simulink model "rocket"  (R2023a)
settings: Solver=ode4  StartTime=0.0  StopTime=t  FixedStep=1/24  RelTol=1e-3
values from neighbouring files (symbols this model uses):
  F_min = F_th / 4    (= 211250)    [rocket_sim.m]
  F_th = 845000    [rocket.m]    (also in rocket_sim.m)
  g = 9.81    [rocket_sim.m]
  h0 = 10000    [rocket.m]    (also in rocket_sim.m)
  h_ref = -1    [rocket_sim.m]
  k = 5.47    [rocket.m]    (also in rocket_sim.m)
  Kd = 1    [rocket.m]    (also in rocket_sim.m = 125000)
  Ki = 1    [rocket.m]    (also in rocket_sim.m = 20000)
  Kp = 1    [rocket.m]    (also in rocket_sim.m = 100000)
  m = 25000    [rocket.m]    (also in rocket_sim.m)
  v_term = -211    [rocket.m]    (also in rocket_sim.m)
settings Model: Creator=eriknymobohne  LastModifiedBy=eriknymobohne

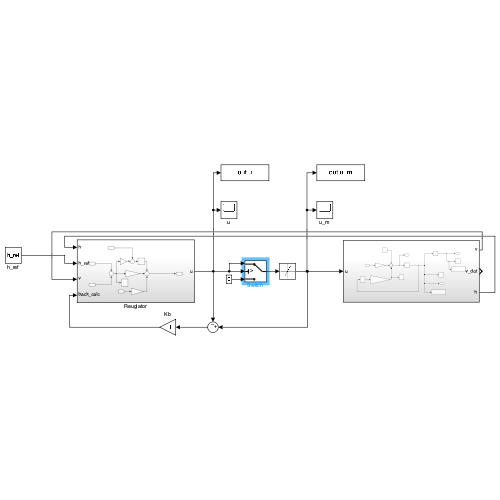
[thumbnail: Simulink's stored preview of the top-level diagram]
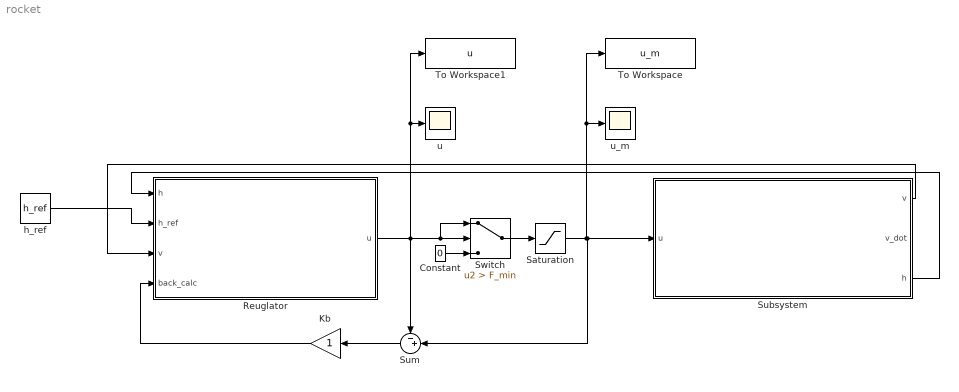
== system rocket ==
  Constant : Constant  Value=0
  Kb : Gain
  Reuglator : Subsystem
  Saturation : Saturate  UpperLimit=F_th  LowerLimit=0
  Subsystem : Subsystem
  Sum : Sum  Inputs=-+|
  Switch : Switch  Criteria=u2 > Threshold  Threshold=F_min  SaturateOnIntegerOverflow=off  InputSameDT=off
  To Workspace : ToWorkspace  VariableName=u_m  SaveFormat=Timeseries  SampleTime=-1
  To Workspace1 : ToWorkspace  VariableName=u  SaveFormat=Timeseries  SampleTime=-1
  h_ref : Constant  Value=h_ref
  u : Scope
  u_m : Scope
  wires:
  h_ref/1 -> Reuglator/2(h_ref)
  Reuglator/1(u) -> Switch/1, Switch/2, To Workspace1/1, u/1, Sum/1
  Saturation/1 -> To Workspace/1, u_m/1, Sum/2, Subsystem/1(u)
  Sum/1 -> Kb/1
  Kb/1 -> Reuglator/4(back_calc)
  Subsystem/3(h) -> Reuglator/1(h)
  Subsystem/1(v) -> Reuglator/3(v)
  Switch/1 -> Saturation/1
  Constant/1 -> Switch/3

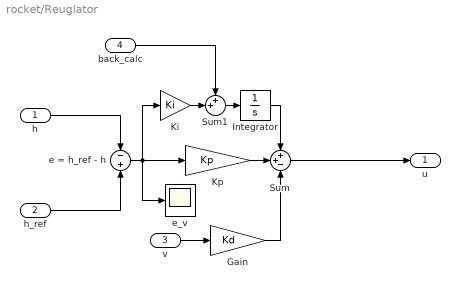
== system rocket/Reuglator ==
  h : Inport
  h_ref : Inport  Port=2
  v : Inport  Port=3
  back_calc : Inport  Port=4
  Gain : Gain  Gain=Kd
  Integrator : Integrator
  Ki : Gain  Gain=Ki
  Kp : Gain  Gain=Kp
  Sum : Sum  Inputs=++-
  Sum1 : Sum  Inputs=++|
  e = h_ref - h : Sum  Inputs=-|+
  e_v : Scope
  u : Outport
  wires:
  h_ref/1 -> e = h_ref - h/2
  h/1 -> e = h_ref - h/1
  e = h_ref - h/1 -> e_v/1, Ki/1, Kp/1
  Kp/1 -> Sum/2
  Integrator/1 -> Sum/1
  v/1 -> Gain/1
  Ki/1 -> Sum1/2
  Sum1/1 -> Integrator/1
  Sum/1 -> u/1
  back_calc/1 -> Sum1/1
  Gain/1 -> Sum/3

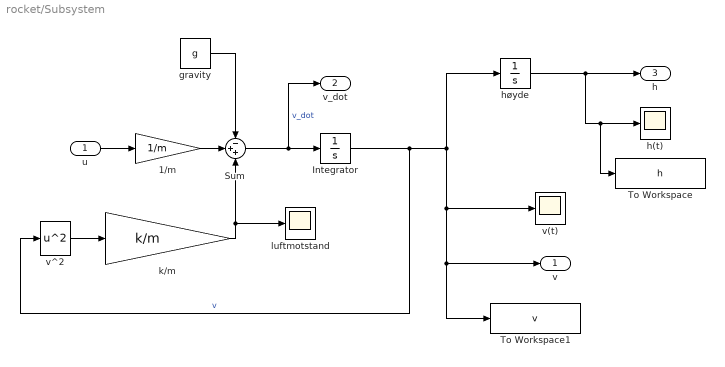
== system rocket/Subsystem ==
  u : Inport
  1/m : Gain  Gain=1/m
  Integrator : Integrator  InitialCondition=v_term
  Sum : Sum  Inputs=-++
  To Workspace : ToWorkspace  VariableName=h  SaveFormat=Timeseries  SampleTime=-1
  To Workspace1 : ToWorkspace  VariableName=v  SaveFormat=Timeseries  SampleTime=-1
  gravity : Constant  Value=g
  h(t) : Scope
  høyde : Integrator  InitialCondition=h0
  k/m : Gain  Gain=k/m
  luftmotstand : Scope
  v(t) : Scope
  v^2 : Math  Operator=square
  v : Outport
  v_dot : Outport  Port=2
  h : Outport  Port=3
  wires:
  Integrator/1 -> v^2/1, høyde/1, v(t)/1, To Workspace1/1, v/1  "v"
  gravity/1 -> Sum/1
  Sum/1 -> v_dot/1, Integrator/1  "v_dot"
  v^2/1 -> k/m/1
  k/m/1 -> luftmotstand/1, Sum/3
  høyde/1 -> h/1, To Workspace/1, h(t)/1
  1/m/1 -> Sum/2
  u/1 -> 1/m/1
